simulink model "Lab4_blocks"  (R2014a)
settings: Solver=ode45  StartTime=0.0  StopTime=10.0  RelTol=1e-3
libraries: simulink x2, dspswit3 x1
settings Model: Creator=reck2  LastModifiedBy=reck2

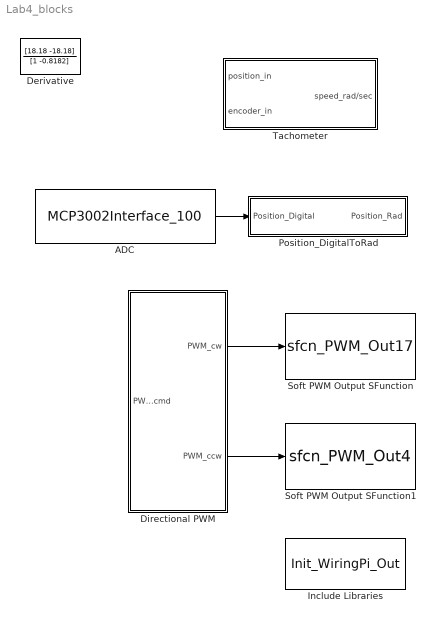
== system Lab4_blocks ==
  ADC : S-Function  InitFcn=try, set_param(gcb,'FunctionName','MCP3002Interface_100'), end  FunctionName=MCP3002Interface_100  SFunctionModules=MCP3002Interface_100_wrapper  EnableBusSupport=off  mask(S-Function Builder){}
      mask help: Simulink:masks:SFunctionBuilder_MD
      mask init:
      | val = [[.9  0.75 0.75 1 1 .9 .9 1]',[1 1 0.75 0.75 .9 .9 1 .9]'];try , sys = get_param(gcb,'SfunBuilderFcnName');if isempty(sys), sys = get_param(gcb,'FunctionName'); end,catch, sys = get_param(gcb,'FunctionName'); end
      settings: CopyFcn=set_param(gcbh,'LinkStatus','none')  PreSaveFcn=try, set_param(gcb,'FunctionName','MCP3002Interface_100'), end  OpenFcn=sfunctionwizard(gcbh)
      mask Display: plot(val(:,1),val(:,2)),disp(sys), port_label('output',1,'y0')
  Derivative : DiscreteFilter  Numerator=[18.18 -18.18]  Denominator=[1 -0.8182]
  Directional PWM : Subsystem
  Include Libraries : S-Function  InitFcn=try, set_param(gcb,'FunctionName','Init_WiringPi_Out'), end  FunctionName=Init_WiringPi_Out  Parameters=uint8(0),uint8(7)  SFunctionModules=Init_WiringPi_Out_wrapper  EnableBusSupport=off  mask(S-Function Builder){}
      mask init: same as Lab4_blocks/ADC
      settings: CopyFcn=set_param(gcbh,'LinkStatus','none')  PreSaveFcn=try, set_param(gcb,'FunctionName','Init_WiringPi_Out'), end  OpenFcn=sfunctionwizard(gcbh)
      mask Display: plot(val(:,1),val(:,2)),disp(sys)
  Position_DigitalToRad : Subsystem
  Soft PWM Output SFunction : S-Function  InitFcn=try, set_param(gcb,'FunctionName','sfcn_PWM_Out17'), end  FunctionName=sfcn_PWM_Out17  Parameters=uint8(0)  SFunctionModules=sfcn_PWM_Out17_wrapper  EnableBusSupport=off  mask(S-Function Builder){}
      mask init: same as Lab4_blocks/ADC
      settings: CopyFcn=set_param(gcbh,'LinkStatus','none')  PreSaveFcn=try, set_param(gcb,'FunctionName','sfcn_PWM_Out17'), end  OpenFcn=sfunctionwizard(gcbh)
      mask Display: plot(val(:,1),val(:,2)),disp(sys), port_label('input',1,'in')
  Soft PWM Output SFunction1 : S-Function  InitFcn=try, set_param(gcb,'FunctionName','sfcn_PWM_Out4'), end  FunctionName=sfcn_PWM_Out4  Parameters=uint8(0)  SFunctionModules=sfcn_PWM_Out4_wrapper  EnableBusSupport=off  mask(S-Function Builder){}
      mask init: same as Lab4_blocks/ADC
      settings: CopyFcn=set_param(gcbh,'LinkStatus','none')  PreSaveFcn=try, set_param(gcb,'FunctionName','sfcn_PWM_Out4'), end  OpenFcn=sfunctionwizard(gcbh)
      mask Display: plot(val(:,1),val(:,2)),disp(sys), port_label('input',1,'in')
  Tachometer : Subsystem
  wires:
  ADC/1 -> Position_DigitalToRad/1(Position_Digital)
  Directional PWM/1(PWM_cw) -> Soft PWM Output SFunction/1
  Directional PWM/2(PWM_ccw) -> Soft PWM Output SFunction1/1

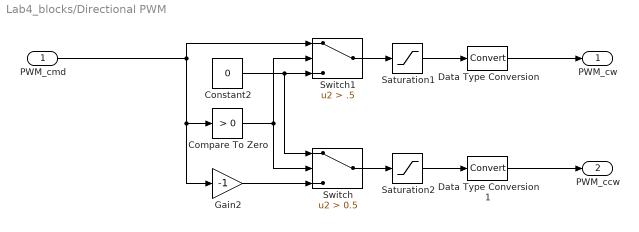
== system Lab4_blocks/Directional PWM ==
  PWM_cmd : Inport
  Compare To Zero : simulink/Logic and Bit Operations/Compare To Zero  relop=>  OutDataTypeStr=boolean
  Constant2 : Constant  Value=0
  Data Type Conversion : DataTypeConversion
  Data Type Conversion1 : DataTypeConversion
  Gain2 : Gain  Gain=-1
  Saturation1 : Saturate  UpperLimit=100  LowerLimit=0
  Saturation2 : Saturate  UpperLimit=100  LowerLimit=0
  Switch : Switch  Criteria=u2 > Threshold  Threshold=0.5
  Switch1 : Switch  Criteria=u2 > Threshold  Threshold=.5
  PWM_cw : Outport
  PWM_ccw : Outport  Port=2
  wires:
  Constant2/1 -> Switch/1, Switch1/3
  Gain2/1 -> Switch/3
  PWM_cmd/1 -> Compare To Zero/1, Gain2/1, Switch1/1
  Data Type Conversion1/1 -> PWM_ccw/1
  Data Type Conversion/1 -> PWM_cw/1
  Saturation2/1 -> Data Type Conversion1/1
  Saturation1/1 -> Data Type Conversion/1
  Compare To Zero/1 -> Switch/2, Switch1/2
  Switch/1 -> Saturation2/1
  Switch1/1 -> Saturation1/1

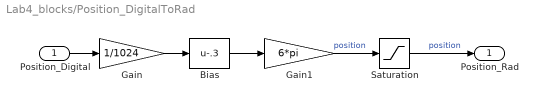
== system Lab4_blocks/Position_DigitalToRad ==
  Position_Digital : Inport
  Bias : Bias  Bias=-.3
  Gain : Gain  Gain=1/1024
  Gain1 : Gain  Gain=6*pi
  Saturation : Saturate  UpperLimit=2*pi+.2  LowerLimit=0
  Position_Rad : Outport
  wires:
  Position_Digital/1 -> Gain/1
  Saturation/1 -> Position_Rad/1  "position"
  Gain1/1 -> Saturation/1  "position"
  Bias/1 -> Gain1/1
  Gain/1 -> Bias/1

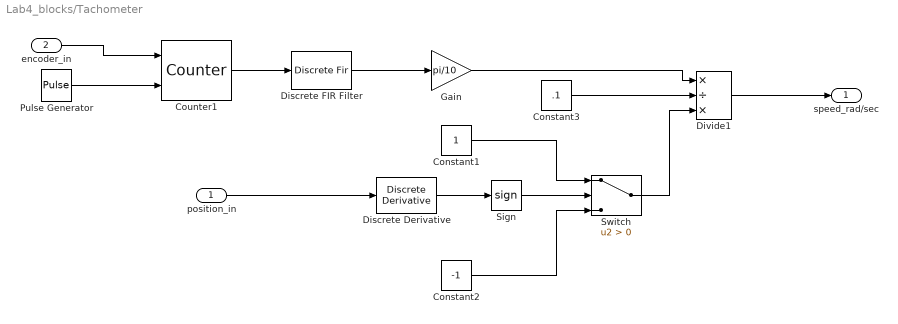
== system Lab4_blocks/Tachometer ==
  position_in : Inport
  encoder_in : Inport  Port=2
  Constant1 : Constant
  Constant2 : Constant  Value=-1
  Constant3 : Constant  Value=.1
  Counter1 : dspswit3/Counter  Direction=Up  CountEvent=Rising edge  CounterSize=User defined  MaxCount=100  InitialCount=0  Output=Count  HitValue=1  ResetInput=on  SamplesPerFrame=1  Ts=1  CntDtype=double  HitDtype=Logical
  Discrete Derivative : simulink/Discrete/Discrete Derivative  gainval=1.0  ICPrevScaledInput=0.0  InputProcessing=Inherited  OutMin=[]  OutMax=[]  OutDataType=fixdt(1, 16)  OutScaling=2^-10  DoSatur=off
  Discrete FIR Filter : DiscreteFir  Coefficients=[0.25 .25 .25 .25]
  Divide1 : Product  Inputs=*/*
  Gain : Gain  Gain=pi/10
  Pulse Generator : DiscretePulseGenerator  PulseType=Time based  Period=.1  PulseWidth=50
  Sign : Signum
  Switch : Switch  Criteria=u2 > Threshold
  speed_rad/sec : Outport
  wires:
  Pulse Generator/1 -> Counter1/2
  Divide1/1 -> speed_rad/sec/1
  Gain/1 -> Divide1/1
  Constant3/1 -> Divide1/2
  Counter1/1 -> Discrete FIR Filter/1
  Constant2/1 -> Switch/3
  Constant1/1 -> Switch/1
  Switch/1 -> Divide1/3
  Sign/1 -> Switch/2
  Discrete Derivative/1 -> Sign/1
  position_in/1 -> Discrete Derivative/1
  encoder_in/1 -> Counter1/1
  Discrete FIR Filter/1 -> Gain/1
